simulink model "RoboBlockRLDO"  (R2021a)
settings: Solver=ode45  StartTime=0.0  StopTime=inf  FixedStep=0.050  RelTol=1e-3
model workspace (MAT data in the model file):
  ANG = 2
  Sig = Simulink.Signal
  Sig.DataType = 'auto'
  Sig.Dimensions = -1
  Sig.DimensionsMode = 'auto'
  Sig.Complexity = 'auto'
  Sig.SampleTime = -1
  Sig.SamplingMode = 'auto'
  Var = 0
  X = 1
  Y = 1
values from neighbouring files (symbols this model uses):
  ang_start = pi/4    (= 0.785398163397)    [ResetFcn.m]
  use_fuzzy = 0    [ResetFcn.m]    (also in createRobotAgent.m = 1)
  x_pos = 3.5    [ResetFcn.m]
  y_pos = 1    [ResetFcn.m]
libraries: simulink x11, fuzblock x2, rllib x2
settings Model: PauseTimes=7  Creator=user  LastModifiedBy=hjcam
settings SolverCC: AlgebraicLoopSolver=TrustRegion
settings DataIOCC: LimitDataPoints=on  SaveFormat=Array  ReturnWorkspaceOutputs=off
settings OptimizationCC: BlockReduction=off  BooleanDataType=off  LifeSpan=inf
settings DebuggingCC: SaveWithParameterizedLinksMsg=none  UnderspecifiedInitializationDetection=Classic  MergeDetectMultiDrivingBlocksExec=none  SignalResolutionControl=TryResolveAllWithWarning  SFUnexpectedBacktrackingDiag=warning  SFNoUnconditionalDefaultTransitionDiag=warning  SFExecutionAtInitializationDiag=none  SFMachineParentedDataDiag=warning  ArithmeticOperatorsInVariantConditions=warning
settings HardwareCC: ProdBitPerPointer=32  ProdBitPerSizeT=32  ProdBitPerPtrDiffT=32  ProdLargestAtomicFloat=None  ProdIntDivRoundTo=Undefined  ProdEndianess=Unspecified  ProdWordSize=32  ProdHWDeviceType=32-bit Generic  TargetUnknown=on
settings ModelReferenceCC: PropagateSignalLabelsOutOfModel=off
settings SFSimCC: SimUseLocalCustomCode=off  CustomCodeUndefinedFunction=UseInterfaceOnly
settings RTWCC: RTWUseLocalCustomCode=off
settings CodeAppCC: StateflowObjectComments=on
settings GRTTargetCC: TargetLangStandard=C89/C90 (ANSI)
settings ConfigComp: CovMetricSettings=dw  CovSaveCumulativeToWorkspaceVar=on  CovSaveSingleToWorkspaceVar=on  CovExternalEMLEnable=off  CovSFcnEnable=off

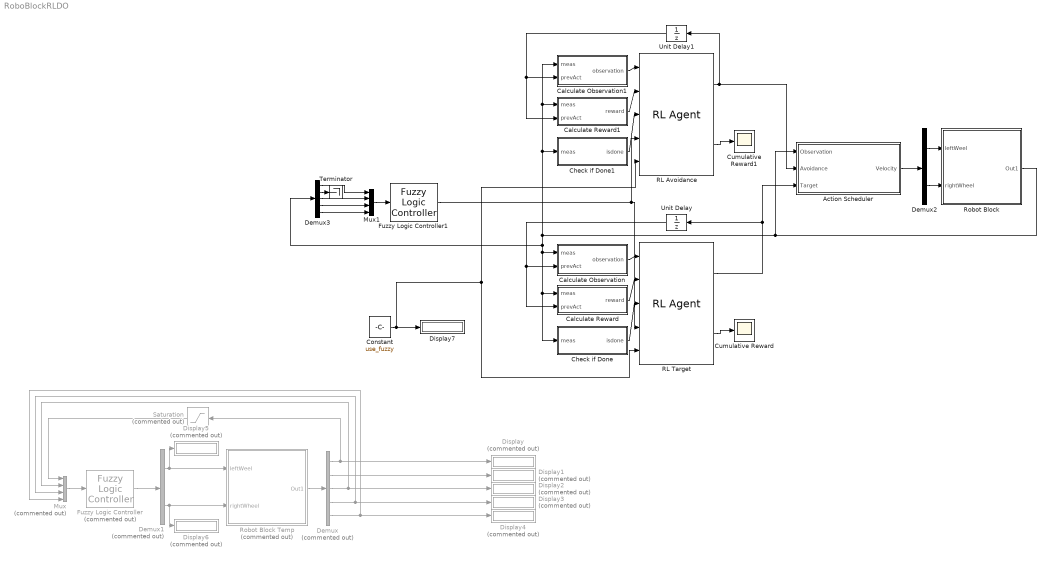
== system RoboBlockRLDO ==
  Action Scheduler : Subsystem
  Calculate Observation : Subsystem
  Calculate Observation1 : Subsystem
  Calculate Reward : Subsystem
  Calculate Reward1 : Subsystem
  Check if Done : Subsystem
  Check if Done1 : Subsystem
  Constant : Constant  Value=use_fuzzy
  Cumulative Reward : Scope
  Cumulative Reward1 : Scope
  Demux : Demux  Commented=on  Outputs=5
  Demux1 : Demux  Commented=on  Outputs=2
  Demux2 : Demux  Outputs=2
  Demux3 : Demux  Outputs=5
  Display{,1..6} (7 alike) : Display  Commented=on
  Display7 : Display
  Fuzzy Logic Controller : fuzblock/Fuzzy Logic  Controller  Commented=on  FIS=robot  OutputSampleNumber=101  DataType=double  FuzzifiedInputs=off  RuleFiringStrengths=off  RuleOutputs=off  AggregatedOutputs=off  SimulateUsing=Interpreted execution  OutOfRangeInputValueMessage=warning  NoRuleFiredMessage=warning  EmptyOutputFuzzySetMessage=warning
  Fuzzy Logic Controller1 : fuzblock/Fuzzy Logic  Controller  FIS=robot  OutputSampleNumber=101  DataType=double  FuzzifiedInputs=off  RuleFiringStrengths=off  RuleOutputs=off  AggregatedOutputs=off  SimulateUsing=Interpreted execution  OutOfRangeInputValueMessage=warning  NoRuleFiredMessage=warning  EmptyOutputFuzzySetMessage=warning
  Mux : Mux  Commented=on
  Mux1 : Mux
  RL Avoidance : rllib/RL Agent  Agent=agentAvoidance  ExternalActionAsInput=on  ProvideCumRwd=on  TreatAsDirectFeedthrough=on
      settings: SourceProductName=Reinforcement Learning
  RL Target : rllib/RL Agent  Agent=agentTarget  ExternalActionAsInput=on  ProvideCumRwd=on  TreatAsDirectFeedthrough=on
      settings: SourceProductName=Reinforcement Learning
  Robot Block : Subsystem  mask(Two-wheel Mobile Robot Model){stID=5013501, modeVal=off, initAngle=ang_start, simStep=0.050, Xpos=x_pos, Ypos=y_pos, isDemo=off}
      mask prompts: stID "Please Enter your UOW student number"; modeVal "Velocity Measurement Mode, select this to disable animations and to allow for the measurement of the velocity of the robot"; initAngle "Set the starting angle (Radians)"; simStep "Override Simulation Step (Defualt is 0.01)"; Xpos "(X,Y)"
      mask help:
      | Robot: Two-wheel robot is driven by two parallel wheels; the speed of each wheel could be set separately
      | Target: target is a single moving point in 2D space
      | Obstacle: obstacle is a group of polygons.
      | Block inputs:
      | vl : velocity of left wheel
      | vr : velocity of right wheel
      | Range of vl, vr: [-2, 2]
      | Block outputs:
      | theta: angle between robot facing and target bearing
      | dis: distance between robot and target
      | ob_loc
      | Range of obstacle detection sensor is 2.5
      | ob_loc=-9	No obstacle detected
      | ob_loc=-2.5	obstacle detected on the front left
      | ob_loc=-5	obstacle detected on the side left
      | ob_loc=0	obstacle detected in the middle
      | ob_loc=2.5	obstacle detected on the front right
      | ob_loc=5	obstacle detected on the side right
      | Battery level/Odometer: total remaining energy/Distance Travelled
      | ultrasonic: a logorithmic signal indicating the distance to the obstacle ( ie 0 = out of sight , a larger number = nearer to the obstacle )
      |
      | The system will crash if the robot collides with the obstacle.
      mask init:
      | stObj.stID = stID;
      | stObj.modeVal = modeVal;
      | stObj.simStep = simStep;
      | stObj.initPos = [Xpos Ypos initAngle];
      | stObj.isDemo = isDemo;
      mask Help:
      | Robot: Two-wheel robot is driven by two parallel wheels; the speed of each wheel could be set separately
      | Target: target is a single moving point in 2D space
      | Obstacle: obstacle is a group of polygons.
      | Block inputs:
      | vl : velocity of left wheel
      | vr : velocity of right wheel
      | Range of vl, vr: [-2, 2]
      | Block outputs:
      | theta: angle between robot facing and target bearing
      | dis: distance between robot and target
      | ob_loc
      | Range of obstacle detection sensor is 2.5
      | ob_loc=-9	No obstacle detected
      | ob_loc=-2.5	obstacle detected on the front left
      | ob_loc=-5	obstacle detected on the side left
      | ob_loc=0	obstacle detected in the middle
      | ob_loc=2.5	obstacle detected on the front right
      | ob_loc=5	obstacle detected on the side right
      | Battery level/Odometer: total remaining energy/Distance Travelled
      | ultrasonic: a logorithmic signal indicating the distance to the obstacle ( ie 0 = out of sight , a larger number = nearer to the obstacle )
      | 
      | The system will crash if the robot collides with the obstacle.
      mask Callback simStep:
      | pm = Simulink.Mask.get(gcb);
      | simStep = pm.getParameter('simStep');
      | set_param(gcs,'FixedStep', simStep.Value);
      mask DialogControl Container4 Prompt: Set the initial starting Coordinates and angle
      mask DialogControl Control3 Prompt: Set starting Position , (must be in the red shaded region)
      mask DialogControl Control3 Callback:
      | [out,~,~,~,~] = roboanimate_org([],[],[],'setup',[]);
      | Xpos = out(1);
      | Ypos = out(2);
      | p = Simulink.Mask.get(gcb);
      | p.Parameters(1,5).set('Value',num2str(Xpos));
      | p.Parameters(1,6).set('Value',num2str(Ypos));
      mask DialogControl Control5 Prompt: Initial Position:
      mask DialogControl Container4_copy Prompt: Run a demo
      mask DialogControl Control2 Prompt: Run  demo
      mask DialogControl Control2 Callback:
      | if(get_param(gcs,'SimulationStatus') == 'stopped')
      | 
      | pm = Simulink.Mask.get(gcb);
      | pm.Parameters(1,7).set('Value','on');
      | options = simset('SrcWorkspace','current');
      | try
      | sim(gcs,[],options)
      | pm.Parameters(1,7).set('Value','off');
      | catch
      | pm.Parameters(1,7).set('Value','off');
      | end
      | 
      | end
      mask Display:
      | patch([ -0.5 0.5 0.5 -0.5],[ -0.5 -0.5 0.5 0.5],[1 1 1])
      | 
      | patch([ -0.2 0.2 0.2 -0.2],[ -0.05 -0.05 0.05 0.05],[0 0 0])
      | 
      | patch(1.1*[ -0.15  0.15 0.15 -0.15],1.1*[ -0.15 -0.15 0.15 0.15],[0 0 0])
      | 
      | patch([ -0.15  0.15 0.15 -0.15],[ -0.15 -0.15 0.15 0.15],[0 0.8 0])
  Robot Block Temp : Subsystem  Commented=on  mask(Two-wheel Mobile Robot Model){stID=5013501, modeVal=off, initAngle=1.696, simStep=0.050, Xpos=4.2582, Ypos=3.4939, isDemo=off}
      mask prompts: stID "Please Enter your UOW student number"; modeVal "Velocity Measurement Mode, select this to disable animations and to allow for the measurement of the velocity of the robot"; initAngle "Set the starting angle (Radians)"; simStep "Override Simulation Step (Defualt is 0.01)"; Xpos "(X,Y)"
      mask help:
      | Robot: Two-wheel robot is driven by two parallel wheels; the speed of each wheel could be set separately
      | Target: target is a single moving point in 2D space
      | Obstacle: obstacle is a group of polygons.
      | Block inputs:
      | vl : velocity of left wheel
      | vr : velocity of right wheel
      | Range of vl, vr: [-2, 2]
      | Block outputs:
      | theta: angle between robot facing and target bearing
      | dis: distance between robot and target
      | ob_loc
      | Range of obstacle detection sensor is 2.5
      | ob_loc=-9	No obstacle detected
      | ob_loc=-2.5	obstacle detected on the front left
      | ob_loc=-5	obstacle detected on the side left
      | ob_loc=0	obstacle detected in the middle
      | ob_loc=2.5	obstacle detected on the front right
      | ob_loc=5	obstacle detected on the side right
      | Battery level/Odometer: total remaining energy/Distance Travelled
      | ultrasonic: a logorithmic signal indicating the distance to the obstacle ( ie 0 = out of sight , a larger number = nearer to the obstacle )
      |
      | The system will crash if the robot collides with the obstacle.
      mask init:
      | stObj.stID = stID;
      | stObj.modeVal = modeVal;
      | stObj.simStep = simStep;
      | stObj.initPos = [Xpos Ypos initAngle];
      | stObj.isDemo = isDemo;
      mask Help:
      | Robot: Two-wheel robot is driven by two parallel wheels; the speed of each wheel could be set separately
      | Target: target is a single moving point in 2D space
      | Obstacle: obstacle is a group of polygons.
      | Block inputs:
      | vl : velocity of left wheel
      | vr : velocity of right wheel
      | Range of vl, vr: [-2, 2]
      | Block outputs:
      | theta: angle between robot facing and target bearing
      | dis: distance between robot and target
      | ob_loc
      | Range of obstacle detection sensor is 2.5
      | ob_loc=-9	No obstacle detected
      | ob_loc=-2.5	obstacle detected on the front left
      | ob_loc=-5	obstacle detected on the side left
      | ob_loc=0	obstacle detected in the middle
      | ob_loc=2.5	obstacle detected on the front right
      | ob_loc=5	obstacle detected on the side right
      | Battery level/Odometer: total remaining energy/Distance Travelled
      | ultrasonic: a logorithmic signal indicating the distance to the obstacle ( ie 0 = out of sight , a larger number = nearer to the obstacle )
      | 
      | The system will crash if the robot collides with the obstacle.
      mask Callback simStep:
      | pm = Simulink.Mask.get(gcb);
      | simStep = pm.getParameter('simStep');
      | set_param(gcs,'FixedStep', simStep.Value);
      mask DialogControl Container4 Prompt: Set the initial starting Coordinates and angle
      mask DialogControl Control3 Prompt: Set starting Position , (must be in the red shaded region)
      mask DialogControl Control3 Callback:
      | [out,~,~,~,~] = roboanimate_org([],[],[],'setup',[]);
      | Xpos = out(1);
      | Ypos = out(2);
      | p = Simulink.Mask.get(gcb);
      | p.Parameters(1,5).set('Value',num2str(Xpos));
      | p.Parameters(1,6).set('Value',num2str(Ypos));
      mask DialogControl Control5 Prompt: Initial Position:
      mask DialogControl Container4_copy Prompt: Run a demo
      mask DialogControl Control2 Prompt: Run  demo
      mask DialogControl Control2 Callback:
      | if(get_param(gcs,'SimulationStatus') == 'stopped')
      | 
      | pm = Simulink.Mask.get(gcb);
      | pm.Parameters(1,7).set('Value','on');
      | options = simset('SrcWorkspace','current');
      | try
      | sim(gcs,[],options)
      | pm.Parameters(1,7).set('Value','off');
      | catch
      | pm.Parameters(1,7).set('Value','off');
      | end
      | 
      | end
      mask Display:
      | patch([ -0.5 0.5 0.5 -0.5],[ -0.5 -0.5 0.5 0.5],[1 1 1])
      | 
      | patch([ -0.2 0.2 0.2 -0.2],[ -0.05 -0.05 0.05 0.05],[0 0 0])
      | 
      | patch(1.1*[ -0.15  0.15 0.15 -0.15],1.1*[ -0.15 -0.15 0.15 0.15],[0 0 0])
      | 
      | patch([ -0.15  0.15 0.15 -0.15],[ -0.15 -0.15 0.15 0.15],[0 0.8 0])
  Saturation : Saturate  Commented=on  UpperLimit=10
  Terminator : Terminator
  Unit Delay : UnitDelay  SampleTime=-1  HasFrameUpgradeWarning=on
  Unit Delay1 : UnitDelay  SampleTime=-1  HasFrameUpgradeWarning=on
  wires:
  Robot Block Temp/1(Out1) -> Demux/1
  Demux/1 -> Saturation/1, Display/1
  Demux/2 -> Display1/1
  Demux/3 -> Mux/2, Display2/1
  Demux/5 -> Mux/4, Display4/1
  Demux1/2 -> Display6/1, Robot Block Temp/2(rightWheel)
  Mux/1 -> Fuzzy Logic Controller/1
  Demux/4 -> Mux/3, Display3/1
  Saturation/1 -> Mux/1
  Demux1/1 -> Robot Block Temp/1(leftWeel), Display5/1
  Fuzzy Logic Controller/1 -> Demux1/1
  RL Target/1 -> Action Scheduler/3(Target), Unit Delay/1
  RL Target/2 -> Cumulative Reward/1
  Calculate Observation/1(observation) -> RL Target/1
  Check if Done/1(isdone) -> RL Target/3
  Unit Delay/1 -> Calculate Reward/2(prevAct), Calculate Observation/2(prevAct)
  Calculate Reward/1(reward) -> RL Target/2
  Unit Delay1/1 -> Calculate Reward1/2(prevAct), Calculate Observation1/2(prevAct)
  Calculate Reward1/1(reward) -> RL Avoidance/2
  RL Avoidance/1 -> Unit Delay1/1, Action Scheduler/2(Avoidance)
  RL Avoidance/2 -> Cumulative Reward1/1
  Calculate Observation1/1(observation) -> RL Avoidance/1
  Check if Done1/1(isdone) -> RL Avoidance/3
  Demux2/1 -> Robot Block/1(leftWeel)
  Demux2/2 -> Robot Block/2(rightWheel)
  Action Scheduler/1(Velocity) -> Demux2/1
  Demux3/5 -> Mux1/4
  Demux3/3 -> Mux1/2
  Demux3/2 -> Terminator/1
  Mux1/1 -> Fuzzy Logic Controller1/1
  Robot Block/1(Out1) -> Action Scheduler/1(Observation), Demux3/1, Check if Done/1(meas), Calculate Reward/1(meas), Calculate Observation/1(meas), Calculate Reward1/1(meas), Calculate Observation1/1(meas), Check if Done1/1(meas)
  Demux3/1 -> Mux1/1
  Demux3/4 -> Mux1/3
  Fuzzy Logic Controller1/1 -> RL Target/4, RL Avoidance/4
  Constant/1 -> RL Target/5, RL Avoidance/5, Display7/1

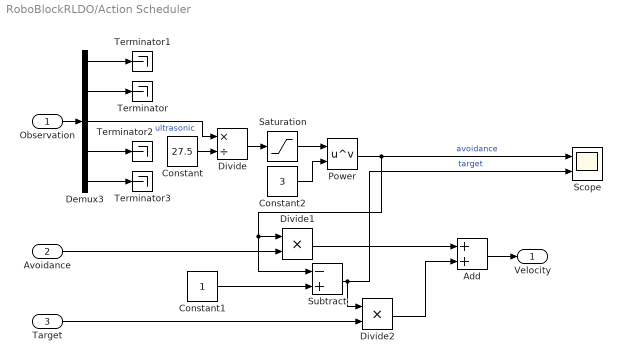
== system RoboBlockRLDO/Action Scheduler ==
  Observation : Inport
  Avoidance : Inport  Port=2
  Target : Inport  Port=3
  Add : Sum
  Constant : Constant  Value=27.5
  Constant1 : Constant
  Constant2 : Constant  Value=3
  Demux3 : Demux  Outputs=5
  Divide : Product  Inputs=*/
  Divide1 : Product  Inputs=**
  Divide2 : Product  Inputs=**
  Power : Math  Operator=pow  SaturateOnIntegerOverflow=on
  Saturation : Saturate  UpperLimit=1  LowerLimit=0
  Scope : Scope  NumInputPorts=2
  Subtract : Sum  Inputs=-+
  Terminator{,1..3} (4 alike) : Terminator
  Velocity : Outport
  wires:
  Demux3/1 -> Terminator1/1
  Demux3/3 -> Divide/1  "ultrasonic"
  Demux3/2 -> Terminator/1
  Demux3/4 -> Terminator2/1
  Observation/1 -> Demux3/1
  Demux3/5 -> Terminator3/1
  Constant/1 -> Divide/2
  Avoidance/1 -> Divide1/2
  Target/1 -> Divide2/2
  Constant1/1 -> Subtract/2
  Subtract/1 -> Scope/2, Divide2/1  "target"
  Divide1/1 -> Add/1
  Divide2/1 -> Add/2
  Add/1 -> Velocity/1
  Divide/1 -> Saturation/1
  Saturation/1 -> Power/1
  Constant2/1 -> Power/2
  Power/1 -> Scope/1, Divide1/1, Subtract/1  "avoidance"

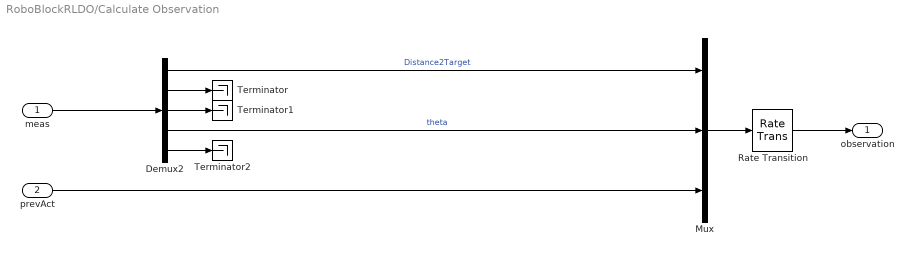
== system RoboBlockRLDO/Calculate Observation ==
  meas : Inport
  prevAct : Inport  Port=2
  Demux2 : Demux  Outputs=5
  Mux : Mux  Inputs=3
  Rate Transition : RateTransition
  Terminator : Terminator
  Terminator1 : Terminator
  Terminator2 : Terminator
  observation : Outport  VectorParamsAs1DForOutWhenUnconnected=off
  wires:
  meas/1 -> Demux2/1
  Mux/1 -> Rate Transition/1
  Rate Transition/1 -> observation/1
  Demux2/1 -> Mux/1  "Distance2Target"
  prevAct/1 -> Mux/3
  Demux2/2 -> Terminator/1
  Demux2/3 -> Terminator1/1
  Demux2/4 -> Mux/2  "theta"
  Demux2/5 -> Terminator2/1

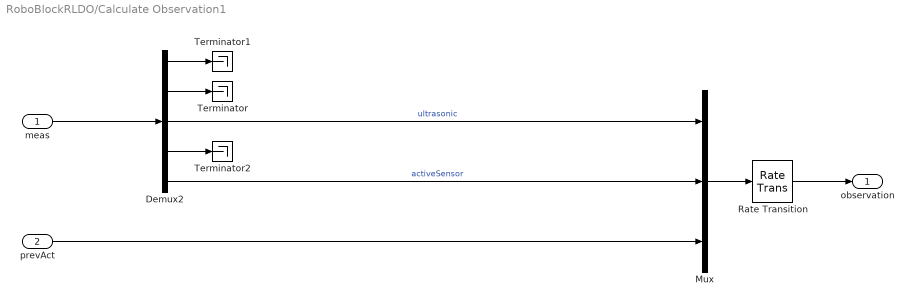
== system RoboBlockRLDO/Calculate Observation1 ==
  meas : Inport
  prevAct : Inport  Port=2
  Demux2 : Demux  Outputs=5
  Mux : Mux  Inputs=3
  Rate Transition : RateTransition
  Terminator : Terminator
  Terminator1 : Terminator
  Terminator2 : Terminator
  observation : Outport  VectorParamsAs1DForOutWhenUnconnected=off
  wires:
  meas/1 -> Demux2/1
  Mux/1 -> Rate Transition/1
  Rate Transition/1 -> observation/1
  prevAct/1 -> Mux/3
  Demux2/2 -> Terminator/1
  Demux2/3 -> Mux/1  "ultrasonic"
  Demux2/4 -> Terminator2/1
  Demux2/5 -> Mux/2  "activeSensor"
  Demux2/1 -> Terminator1/1

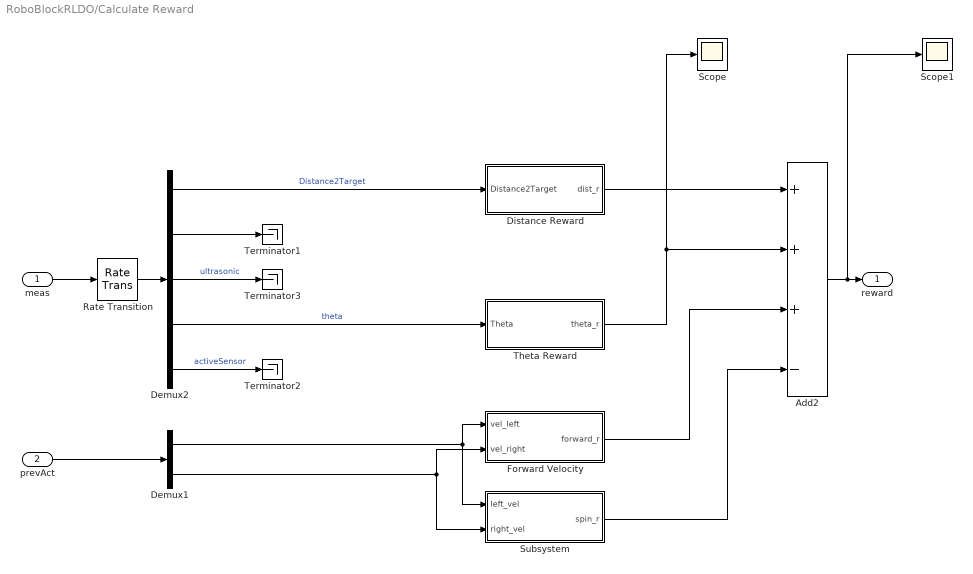
== system RoboBlockRLDO/Calculate Reward ==
  meas : Inport
  prevAct : Inport  Port=2
  Add2 : Sum  Inputs=+++-
  Demux1 : Demux  Outputs=2
  Demux2 : Demux  Outputs=5
  Distance Reward : Subsystem
  Forward Velocity : Subsystem
  Rate Transition : RateTransition  OutPortSampleTime=Ts
  Scope : Scope
  Scope1 : Scope
  Subsystem : Subsystem
  Terminator1 : Terminator
  Terminator2 : Terminator
  Terminator3 : Terminator
  Theta Reward : Subsystem
  reward : Outport  VectorParamsAs1DForOutWhenUnconnected=off
  wires:
  meas/1 -> Rate Transition/1
  Add2/1 -> Scope1/1, reward/1
  Demux2/5 -> Terminator2/1  "activeSensor"
  Rate Transition/1 -> Demux2/1
  Demux2/4 -> Theta Reward/1(Theta)  "theta"
  Demux1/1 -> Subsystem/1(left_vel), Forward Velocity/1(vel_left)
  Demux1/2 -> Subsystem/2(right_vel), Forward Velocity/2(vel_right)
  Distance Reward/1(dist_r) -> Add2/1
  Demux2/1 -> Distance Reward/1(Distance2Target)  "Distance2Target"
  Demux2/2 -> Terminator1/1
  Demux2/3 -> Terminator3/1  "ultrasonic"
  prevAct/1 -> Demux1/1
  Theta Reward/1(theta_r) -> Add2/2, Scope/1
  Forward Velocity/1(forward_r) -> Add2/3
  Subsystem/1(spin_r) -> Add2/4

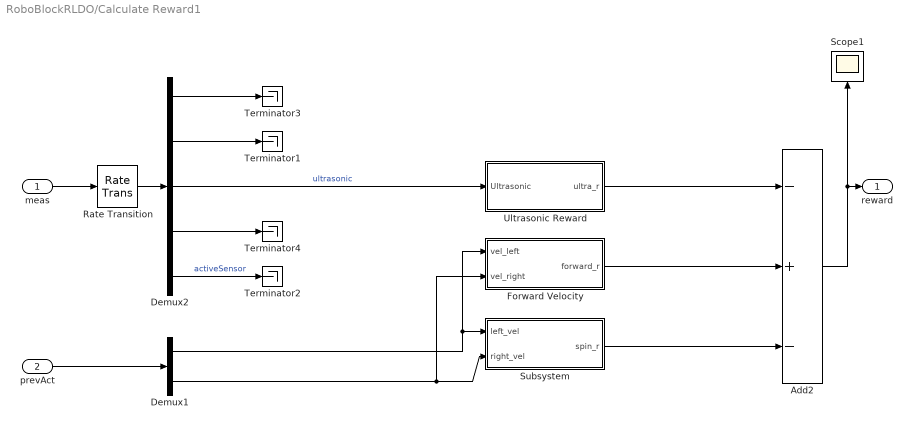
== system RoboBlockRLDO/Calculate Reward1 ==
  meas : Inport
  prevAct : Inport  Port=2
  Add2 : Sum  Inputs=-+-
  Demux1 : Demux  Outputs=2
  Demux2 : Demux  Outputs=5
  Forward Velocity : Subsystem
  Rate Transition : RateTransition  OutPortSampleTime=Ts
  Scope1 : Scope
  Subsystem : Subsystem
  Terminator{1..4} (4 alike) : Terminator
  Ultrasonic Reward : Subsystem
  reward : Outport  VectorParamsAs1DForOutWhenUnconnected=off
  wires:
  meas/1 -> Rate Transition/1
  Add2/1 -> Scope1/1, reward/1
  Demux2/5 -> Terminator2/1  "activeSensor"
  Rate Transition/1 -> Demux2/1
  Demux2/4 -> Terminator4/1
  Ultrasonic Reward/1(ultra_r) -> Add2/1
  Demux1/1 -> Subsystem/1(left_vel), Forward Velocity/1(vel_left)
  Demux1/2 -> Forward Velocity/2(vel_right), Subsystem/2(right_vel)
  Demux2/1 -> Terminator3/1
  Demux2/2 -> Terminator1/1
  Demux2/3 -> Ultrasonic Reward/1(Ultrasonic)  "ultrasonic"
  prevAct/1 -> Demux1/1
  Forward Velocity/1(forward_r) -> Add2/2
  Subsystem/1(spin_r) -> Add2/3

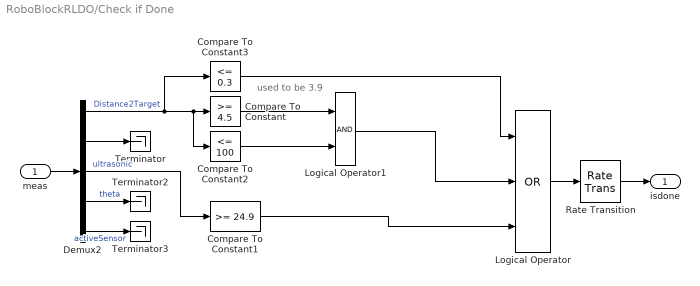
== system RoboBlockRLDO/Check if Done ==
  note: used to be 3.9
  meas : Inport
  Compare To Constant : simulink/Logic and Bit Operations/Compare To Constant  relop=>=  const=4.5  OutDataTypeStr=boolean
  Compare To Constant1 : simulink/Logic and Bit Operations/Compare To Constant  relop=>=  const=24.9  OutDataTypeStr=boolean
  Compare To Constant2 : simulink/Logic and Bit Operations/Compare To Constant  relop=<=  const=100  OutDataTypeStr=boolean
  Compare To Constant3 : simulink/Logic and Bit Operations/Compare To Constant  relop=<=  const=0.3  OutDataTypeStr=boolean
  Demux2 : Demux  Outputs=5
  Logical Operator : Logic  Operator=OR  Inputs=3  AllPortsSameDT=off  OutDataTypeStr=boolean
  Logical Operator1 : Logic  AllPortsSameDT=off  OutDataTypeStr=boolean
  Rate Transition : RateTransition
  Terminator : Terminator
  Terminator2 : Terminator
  Terminator3 : Terminator
  isdone : Outport  VectorParamsAs1DForOutWhenUnconnected=off
  wires:
  Logical Operator/1 -> Rate Transition/1
  Rate Transition/1 -> isdone/1
  Demux2/5 -> Terminator3/1  "activeSensor"
  Demux2/2 -> Terminator/1
  Demux2/3 -> Compare To Constant1/1  "ultrasonic"
  Demux2/1 -> Compare To Constant3/1, Compare To Constant2/1, Compare To Constant/1  "Distance2Target"
  meas/1 -> Demux2/1
  Demux2/4 -> Terminator2/1  "theta"
  Compare To Constant/1 -> Logical Operator1/1
  Compare To Constant2/1 -> Logical Operator1/2
  Compare To Constant1/1 -> Logical Operator/3
  Logical Operator1/1 -> Logical Operator/2
  Compare To Constant3/1 -> Logical Operator/1

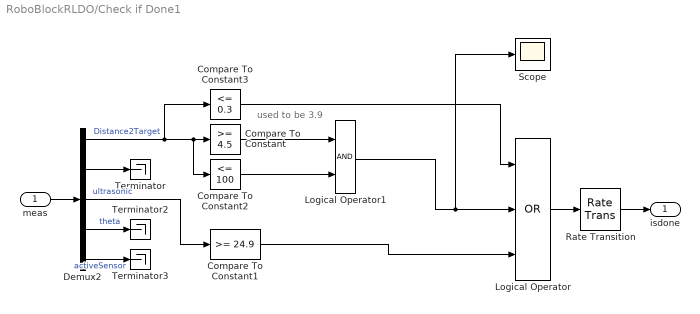
== system RoboBlockRLDO/Check if Done1 ==
  note: used to be 3.9
  meas : Inport
  Compare To Constant : simulink/Logic and Bit Operations/Compare To Constant  relop=>=  const=4.5  OutDataTypeStr=boolean
  Compare To Constant1 : simulink/Logic and Bit Operations/Compare To Constant  relop=>=  const=24.9  OutDataTypeStr=boolean
  Compare To Constant2 : simulink/Logic and Bit Operations/Compare To Constant  relop=<=  const=100  OutDataTypeStr=boolean
  Compare To Constant3 : simulink/Logic and Bit Operations/Compare To Constant  relop=<=  const=0.3  OutDataTypeStr=boolean
  Demux2 : Demux  Outputs=5
  Logical Operator : Logic  Operator=OR  Inputs=3  AllPortsSameDT=off  OutDataTypeStr=boolean
  Logical Operator1 : Logic  AllPortsSameDT=off  OutDataTypeStr=boolean
  Rate Transition : RateTransition
  Scope : Scope
  Terminator : Terminator
  Terminator2 : Terminator
  Terminator3 : Terminator
  isdone : Outport  VectorParamsAs1DForOutWhenUnconnected=off
  wires:
  Logical Operator/1 -> Rate Transition/1
  Rate Transition/1 -> isdone/1
  Demux2/5 -> Terminator3/1  "activeSensor"
  Demux2/2 -> Terminator/1
  Demux2/3 -> Compare To Constant1/1  "ultrasonic"
  Demux2/1 -> Compare To Constant3/1, Compare To Constant2/1, Compare To Constant/1  "Distance2Target"
  meas/1 -> Demux2/1
  Demux2/4 -> Terminator2/1  "theta"
  Compare To Constant/1 -> Logical Operator1/1
  Compare To Constant2/1 -> Logical Operator1/2
  Compare To Constant1/1 -> Logical Operator/3
  Logical Operator1/1 -> Scope/1, Logical Operator/2
  Compare To Constant3/1 -> Logical Operator/1

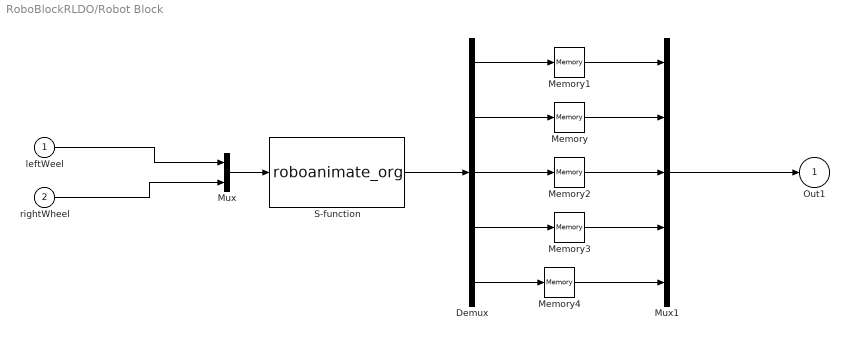
== system RoboBlockRLDO/Robot Block ==
  leftWeel : Inport
  rightWheel : Inport  Port=2
  Demux : Demux  Outputs=5
  Memory{,2..4} (4 alike) : Memory
  Memory1 : Memory  InitialCondition=1000
  Mux : Mux  Inputs=2
  Mux1 : Mux  Inputs=5
  S-function : S-Function  FunctionName=roboanimate_org  Parameters=stObj  SFunctionDeploymentMode=off  EnableBusSupport=off
  Out1 : Outport
  wires:
  rightWheel/1 -> Mux/2
  leftWeel/1 -> Mux/1
  Mux/1 -> S-function/1
  S-function/1 -> Demux/1
  Memory1/1 -> Mux1/1
  Demux/1 -> Memory1/1
  Memory/1 -> Mux1/2
  Memory2/1 -> Mux1/3
  Demux/3 -> Memory2/1
  Demux/2 -> Memory/1
  Demux/4 -> Memory3/1
  Memory3/1 -> Mux1/4
  Demux/5 -> Memory4/1
  Memory4/1 -> Mux1/5
  Mux1/1 -> Out1/1

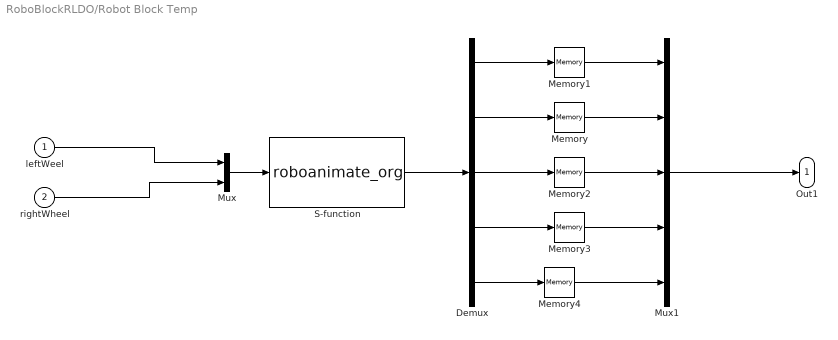
== system RoboBlockRLDO/Robot Block Temp ==
  leftWeel : Inport
  rightWheel : Inport  Port=2
  Demux : Demux  Outputs=5
  Memory{,2..4} (4 alike) : Memory
  Memory1 : Memory  InitialCondition=1000
  Mux : Mux  Inputs=2
  Mux1 : Mux  Inputs=5
  S-function : S-Function  FunctionName=roboanimate_org  Parameters=stObj  SFunctionDeploymentMode=off  EnableBusSupport=off
  Out1 : Outport
  wires:
  rightWheel/1 -> Mux/2
  leftWeel/1 -> Mux/1
  Mux/1 -> S-function/1
  S-function/1 -> Demux/1
  Memory1/1 -> Mux1/1
  Demux/1 -> Memory1/1
  Memory/1 -> Mux1/2
  Memory2/1 -> Mux1/3
  Demux/3 -> Memory2/1
  Demux/2 -> Memory/1
  Demux/4 -> Memory3/1
  Memory3/1 -> Mux1/4
  Demux/5 -> Memory4/1
  Memory4/1 -> Mux1/5
  Mux1/1 -> Out1/1

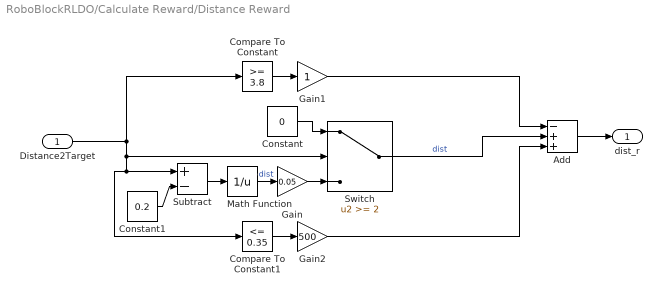
== system RoboBlockRLDO/Calculate Reward/Distance Reward ==
  Distance2Target : Inport
  Add : Sum  Inputs=-++
  Compare To Constant : simulink/Logic and Bit Operations/Compare To Constant  relop=>=  const=3.8  OutDataTypeStr=boolean
  Compare To Constant1 : simulink/Logic and Bit Operations/Compare To Constant  relop=<=  const=0.35  OutDataTypeStr=boolean
  Constant : Constant  Value=0
  Constant1 : Constant  Value=0.2
  Gain : Gain  Gain=0.05
  Gain1 : Gain
  Gain2 : Gain  Gain=500
  Math Function : Math  Operator=reciprocal  SaturateOnIntegerOverflow=on
  Subtract : Sum  Inputs=+-
  Switch : Switch  Threshold=2
  dist_r : Outport
  wires:
  Distance2Target/1 -> Switch/2, Subtract/1, Compare To Constant1/1, Compare To Constant/1
  Switch/1 -> Add/2  "dist"
  Compare To Constant/1 -> Gain1/1
  Add/1 -> dist_r/1
  Constant/1 -> Switch/1
  Gain/1 -> Switch/3
  Gain1/1 -> Add/1
  Compare To Constant1/1 -> Gain2/1
  Gain2/1 -> Add/3
  Constant1/1 -> Subtract/2
  Math Function/1 -> Gain/1  "dist"
  Subtract/1 -> Math Function/1

== system RoboBlockRLDO/Calculate Reward/Forward Velocity ==
  vel_left : Inport
  vel_right : Inport  Port=2
  Add1 : Sum
  Forward : Gain  Gain=0.025
  forward_r : Outport
  wires:
  vel_left/1 -> Add1/1
  Add1/1 -> Forward/1
  Forward/1 -> forward_r/1
  vel_right/1 -> Add1/2

== system RoboBlockRLDO/Calculate Reward/Subsystem ==
  left_vel : Inport
  right_vel : Inport  Port=2
  Abs : Abs
  Add3 : Sum  Inputs=+-
  Spin : Gain  Gain=0.025
  Square : Math  Operator=square  SignedPower=on  RndMeth=Zero  SaturateOnIntegerOverflow=on
  spin_r : Outport
  wires:
  Abs/1 -> Square/1
  Spin/1 -> spin_r/1
  Square/1 -> Spin/1
  Add3/1 -> Abs/1
  right_vel/1 -> Add3/2
  left_vel/1 -> Add3/1

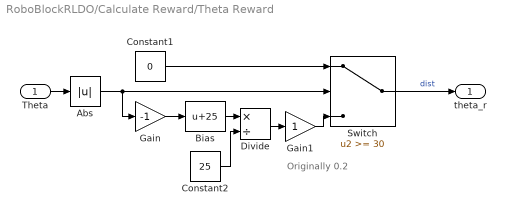
== system RoboBlockRLDO/Calculate Reward/Theta Reward ==
  note: Originally 0.2
  Theta : Inport
  Abs : Abs
  Bias : Bias  Bias=25
  Constant1 : Constant  Value=0
  Constant2 : Constant  Value=25
  Divide : Product  Inputs=*/
  Gain : Gain  Gain=-1
  Gain1 : Gain
  Switch : Switch  Threshold=30
  theta_r : Outport
  wires:
  Theta/1 -> Abs/1
  Abs/1 -> Gain/1, Switch/2
  Constant1/1 -> Switch/1
  Gain/1 -> Bias/1
  Bias/1 -> Divide/1
  Constant2/1 -> Divide/2
  Divide/1 -> Gain1/1
  Gain1/1 -> Switch/3
  Switch/1 -> theta_r/1  "dist"

== system RoboBlockRLDO/Calculate Reward1/Forward Velocity ==
  vel_left : Inport
  vel_right : Inport  Port=2
  Add1 : Sum
  Forward : Gain  Gain=0.01
  forward_r : Outport
  wires:
  vel_left/1 -> Add1/1
  Add1/1 -> Forward/1
  Forward/1 -> forward_r/1
  vel_right/1 -> Add1/2

== system RoboBlockRLDO/Calculate Reward1/Subsystem ==
  left_vel : Inport
  right_vel : Inport  Port=2
  Abs : Abs
  Add3 : Sum  Inputs=+-
  Spin : Gain  Gain=0.025
  Square : Math  Operator=square  SignedPower=on  RndMeth=Zero  SaturateOnIntegerOverflow=on
  spin_r : Outport
  wires:
  Abs/1 -> Square/1
  Spin/1 -> spin_r/1
  Square/1 -> Spin/1
  Add3/1 -> Abs/1
  right_vel/1 -> Add3/2
  left_vel/1 -> Add3/1

== system RoboBlockRLDO/Calculate Reward1/Ultrasonic Reward ==
  note: Was originally 25
  Ultrasonic : Inport
  Compare To Constant1 : simulink/Logic and Bit Operations/Compare To Constant  relop=>=  const=24.85  OutDataTypeStr=boolean
  Gain : Gain  Gain=25
  ultra_r : Outport
  wires:
  Ultrasonic/1 -> Compare To Constant1/1
  Compare To Constant1/1 -> Gain/1
  Gain/1 -> ultra_r/1
